simulink model "EV_powertrain"  (R2020a)
settings: Solver=FixedStepAuto  StartTime=0.0  StopTime=120.0  RelTol=1e-3
values from neighbouring files (symbols this model uses):
  A = 1452*mm*1799*mm    (= 2.612148)    [Model_parameters.m]
  b_r = 4.924e-4*(Nm/rad)    (= 0.0004924)    [Model_parameters.m]
  C_d = 0.27    [Model_parameters.m]
  c_roll = 0.0125    [Model_parameters.m]
  g = 9.81*(meters/(sec^2))    (= 9.81)    [Model_parameters.m]
  J_r = 0.089*kg*meters^2    (= 0.089)    [Model_parameters.m]
  K_rg = 10^13*(Newton/meters)    (= 10000000000000)    [Model_parameters.m]
  lambda_pm = 0.1039*Weber    (= 0.1039)    [Model_parameters.m]
  M = 1300*kg    (= 1300)    [Model_parameters.m]
  P_2_0 = 0    [Model_parameters.m]
  P_4_0 = 0    [Model_parameters.m]
  pp = 4    [Model_parameters.m]
  pwm_switch_period = 2e-5    (= 2e-05)    [Model_parameters.m]
  r_g = 9.7*r_r    (= 0.097)    [Model_parameters.m]
  r_r = 1*cm    (= 0.01)    [Model_parameters.m]
  r_w = 32*cm    (= 0.32)    [Model_parameters.m]
  rho = 1.225*(kg/(meters^3))    (= 1.225)    [Model_parameters.m]
  slope_out = tan(-0.3*[ 0  0  0  0  0  0  0  0  0  0 0]*degrees)    [Model_parameters.m]
  x_5_0 = 0    [Model_parameters.m]
  x_in = [ 0 12 38 65 78 100 112 138 165 178 200]*meters    [Model_parameters.m]
libraries: eePwmGenerator x3, simulink x1, autolibdatasheetbattery x1, autolibmotorctrlr x1, autolibpmsmexterior x1, autolibinverter x1
settings Model: Creator=giaco  LastModifiedBy=annac

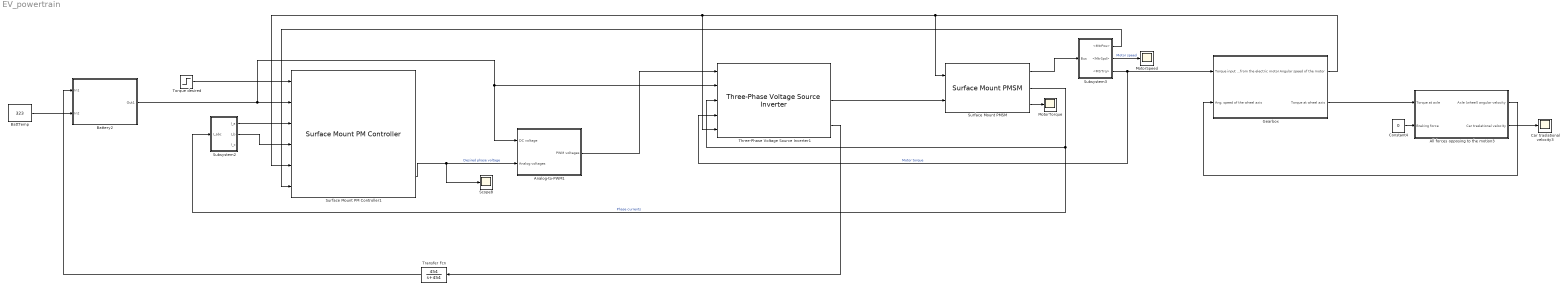
== system EV_powertrain ==
  All forces opposing to the motion3 : Subsystem
  Analog-to-PWM1 : Subsystem
  BattTemp : Constant  Value=323
  Battery2 : Subsystem
  Car traslational velocity3 : Scope
  Constant4 : Constant  Value=0
  Gearbox : Subsystem
  MotorSpeed : Scope
  MotorTorque : Scope
  Scope8 : Scope
  Subsystem2 : Subsystem
  Subsystem3 : Subsystem
  Surface Mount PM Controller1 : autolibmotorctrlr/Surface Mount PM Controller  control_type=Torque Control  Rs=R_s  Ldq=L_s  Ld=0.000391  Lq=0.000391  lambda_pm=lambda_pm  PolePairs=pp  Mechanical=[J_r, b_r, 0]  T_max=max_torque_motor  bp=10  T_mtpa=[0 6.66669841797461 13.3335873347246 20.0008572036754 26.6686983876046 33.3373011134498 40.0068554272732 46.6775511494351 53.3495778300274 60.0231247046184]  id_mtpa=[0 -0.0287202961052195 -0.114874619738106 -0.258443284350566 -0.459393504010068 -0.717679430800711 -1.03324220704656 -1.40601003221657 -1.8358982443354 -2.32280941568585]  iq_mtpa=[0 9.30574388067393 18.6112218818157 27.9161683137524 37.220317866163 46.5234057968387 55.8251681193482 65.12534178925 74.4236648884977 83.7198768076925]  idq_limits=401.0266  EV_current=500000  Tst=T_sample_torque_control  Kp_d=1178.7256  Kp_q=1178.7256  Ki=628318.5307  EV_motion=[20, 4, 0.8]  EV_sf=100  ba=50  Ksa=10  Kisa=0.05  Ksf=10  Jcomp=J_r  Fv=b_r  Fs=0  param_loss=Single efficiency measurement  eff=inverter_efficiency  w_loss_bp=[0 200 400 600 800 1000]  T_loss_bp=[0 25 50 75 100]  losses_table=[100 100 100 100 100;100 150 200 250 300;100 200 300 400 500;100 250 400 550 700;100 300 500 700 900;100 350 600 850 1100]  w_eff_bp=[200 400 600 800 1000]  T_eff_bp=[25 50 75 100]  efficiency_table=[96.2 98.1 98.7 99;98.1 99 99.4 99.5;98.7 99.4 99.6 99.7;99 99.5 99.7 99.8;99.2 99.6 99.7 99.8]  x_w_bp=[-1000 -800 -600 -400 -200 200 400 600 800 1000]  x_T_bp=[-100 -75 -50 -25 25 50 75 100]  x_losses_mat=[200.400801603196 225.67703109328 200.803212851408 201.612903225806 199.999999999997 200 225 200;160.320641282556 180.541624874624 201.005025125625 202.020202020203 200 200 180 160;180.541624874624 180.722891566267 181.086519114686 197.568389057748 194.999999999999 179.999999999997 180 180;201.005025125625 181.086519114686 202.020202020203 193.67991845056 190 200 179.999999999997 200;202.020202020203 197.568389057748 193.67991845056 197.505197505197 190 190 194.999999999999 200;200 194.999999999999 190 190 197.505197505197 193.67991845056 197.568389057748 202.020202020203;200 179.999999999997 200 190 193.67991845056 202.020202020203 181.086519114686 201.005025125625;180 180 179.999999999997 194.999999999999 197.568389057748 181.086519114686 180.722891566267 180.541624874624;160 180 200 200 202.020202020203 201.005025125625 180.541624874624 160.320641282556;200 225 200 199.999999999997 201.612903225806 200.803212851408 225.67703109328 200.400801603196]  Tsm=5e-4
      settings: SourceProductBaseCode=PW
  Surface Mount PMSM : autolibpmsmexterior/Surface Mount PMSM  port_config=Speed  sim_type=Continuous  Ts=0.001  FilePath=E:\Sandbox\Bauto\Work\surfacepmsm_motordata.m  P=pp  Rs=R_s  Ldq_=L_s  KConstText=Permanent flux linkage constant (lambda_pm):  lambda_pm=lambda_pm  Ke=159.9771  Kt=1.323  mechanical=[0.0027, 4.924e-4, 0]  idq0=[0 0]  theta_init=0  omega_init=0  KConst=lambda_pm  lambda_pm_calc=lambda_pm  RefBlkName='autolibpmsmexterior/Surface Mount PMSM'  aMode=1  Ldq="[0.000391    0.000391]"
      settings: SourceProductBaseCode=PW,MT,VE,VP
  Three-Phase Voltage Source Inverter1 : autolibinverter/Three-Phase Voltage Source Inverter  InvrtrTmpInpEnbl=off  enable_hdl=off  model_type=Switch inputs  fs=10000  w_eff_bp=[-1000 -500 0 500 1000]  n1=128  T_eff_bp=[-200 -100 0 100 200]  Temp_eff_bp=[213.15 293.15 373.15]  n2=128  ploss_table=[1 0.999 0.989 0.997 0.996;0.995 0.994 0.993 0.992 0.991;0.990 0.989 0.988 0.987 0.986;0.985 0.984 0.983 0.982 0.981;0.980 0.979 0.978 0.977 0.976]  ploss_table_3d=cat(3,0.95*[1 0.999 0.989 0.997 0.996;0.995 0.994 0.993 0.992 0.991;0.990 0.989 0.988 0.987 0.986;0.985 0.984 0.983 0.982 0.981;0.980 0.979 0.978 0.977 0.976],[1 0.999 0.989 0.997 0.996;0.995 0.994 0.993 0.992 0.991;0.990 0.989 0.988 0.987 0.986;0.985 0.984 0.983 0.982 0.981;0.980 0.979 0.978 0.977 0.976],0.92*[1 0.999 0.989 0.997 0.996;0.995 0.994 0.993 0.992 0.991;0.990 0.989 0.988 0.987 0.986;0.985 0.984 0.983 0.982 0.981;0.980 0.979 0.978 0.977 0.976])  preExtrapFlag=off  u1max=1000  u1min=-1000  u2max=200  u2min=-200  intPrec=23  RefBlkName='autolibmappedmotor/Mapped Motor'  CalLossMapData={'BaseCageProjectFileName','';'BaseMbcProjectFileName','';'TaskName','Calibrate Inverter Loss Map';'ChildTasks',{{'DataName','';'TaskName','Import Loss Data'},{'TaskName','Generate Response Models'},{'TaskName','Generate Calibration'},{'TaskName','Update Block Parameters'}}}  CalLossWithTempMapData={}
      settings: SourceProductBaseCode=PW,MT,VE,VP
  Torque desired : Step  Time=0.2  After=200  SampleTime=0
  Transfer Fcn : TransferFcn  Numerator=[454]  Denominator=[1 454]
  wires:
  Surface Mount PM Controller1/3 -> Scope8/1, Analog-to-PWM1/2(Analog voltages)  "Desired phase voltage"
  Torque desired/1 -> Surface Mount PM Controller1/1
  Analog-to-PWM1/1(PWM voltages) -> Three-Phase Voltage Source Inverter1/1
  Battery2/1(Out1) -> Analog-to-PWM1/1(DC voltage), Three-Phase Voltage Source Inverter1/2, Surface Mount PM Controller1/2
  Surface Mount PMSM/2 -> Three-Phase Voltage Source Inverter1/3, Subsystem2/1(I_abc)  "Phase currents"
  Surface Mount PMSM/1 -> Subsystem3/1(Bus)
  Subsystem3/3(<MtrTrq>) -> Gearbox/1(Torque input from the electric motor), Three-Phase Voltage Source Inverter1/4  "Motor torque"
  Three-Phase Voltage Source Inverter1/2 -> Surface Mount PMSM/2
  Subsystem3/1(<MtrPos>) -> Surface Mount PM Controller1/6
  Subsystem2/1(I_a) -> Surface Mount PM Controller1/3
  Subsystem2/2(I_b) -> Surface Mount PM Controller1/4
  Gearbox/1(Angular speed of the motor) -> Surface Mount PMSM/1, Three-Phase Voltage Source Inverter1/5, Surface Mount PM Controller1/5
  Constant4/1 -> All forces opposing to the motion3/2(Braking force)
  All forces opposing to the motion3/2(Car traslational velocity) -> Car traslational velocity3/1
  Gearbox/2(Torque at wheel axis) -> All forces opposing to the motion3/1(Torque at axle)
  All forces opposing to the motion3/1(Axle (wheel) angular velocity) -> Gearbox/2(Ang. speed of the wheel axis)
  BattTemp/1 -> Battery2/2(In2)
  Three-Phase Voltage Source Inverter1/3 -> Transfer Fcn/1
  Transfer Fcn/1 -> Battery2/1(In1)
  Surface Mount PMSM/3 -> MotorTorque/1
  Subsystem3/2(<MtrSpd>) -> MotorSpeed/1  "Motor speed"

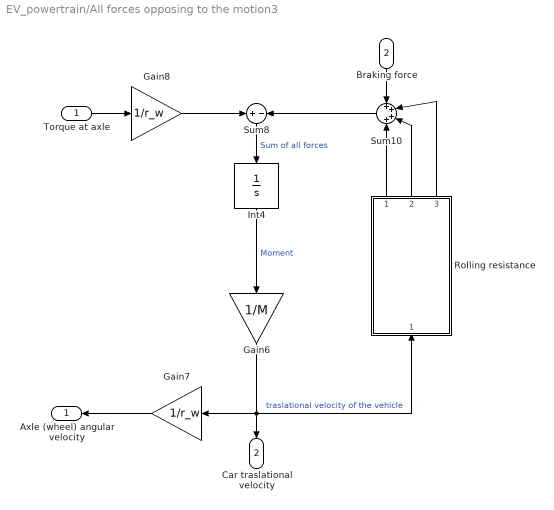
== system EV_powertrain/All forces opposing to the motion3 ==
  Torque at axle : Inport
  Braking force : Inport  Port=2
  Gain6 : Gain  Gain=1/M  SaturateOnIntegerOverflow=on  OutDataTypeStr=Inherit: Same as input  ParamDataTypeStr=Inherit: Same as input
  Gain7 : Gain  Gain=1/r_w  SaturateOnIntegerOverflow=on  OutDataTypeStr=Inherit: Same as input  ParamDataTypeStr=Inherit: Same as input
  Gain8 : Gain  Gain=1/r_w  SaturateOnIntegerOverflow=on  OutDataTypeStr=Inherit: Same as input  ParamDataTypeStr=Inherit: Same as input
  Int4 : Integrator  InitialCondition=P_4_0
  Rolling resistance : Subsystem
  Sum10 : Sum  Inputs=++++  InputSameDT=on  SaturateOnIntegerOverflow=on  OutDataTypeStr=Inherit: Same as first input
  Sum8 : Sum  Inputs=+|-  InputSameDT=on  SaturateOnIntegerOverflow=on  OutDataTypeStr=Inherit: Same as first input
  Axle (wheel) angular velocity : Outport  VectorParamsAs1DForOutWhenUnconnected=off
  Car traslational velocity : Outport  Port=2  VectorParamsAs1DForOutWhenUnconnected=off
  wires:
  Gain7/1 -> Axle (wheel) angular velocity/1
  Gain8/1 -> Sum8/1
  Sum8/1 -> Int4/1  "Sum of all forces"
  Gain6/1 -> Gain7/1, Rolling resistance/1(Traslational velocity), Car traslational velocity/1  "traslational velocity of the vehicle"
  Int4/1 -> Gain6/1  "Moment"
  Sum10/1 -> Sum8/2
  Torque at axle/1 -> Gain8/1
  Braking force/1 -> Sum10/1
  Rolling resistance/1(Rolling res) -> Sum10/4
  Rolling resistance/2("  Road slope") -> Sum10/3
  Rolling resistance/3(" Drag Force") -> Sum10/2

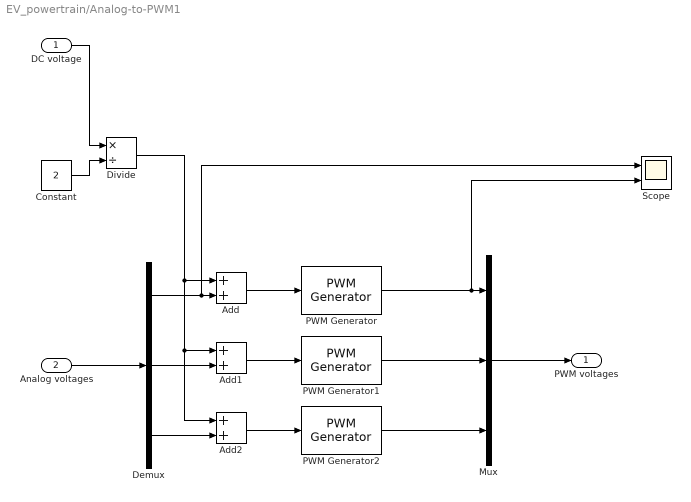
== system EV_powertrain/Analog-to-PWM1 ==
  DC voltage : Inport
  Analog voltages : Inport  Port=2
  Add : Sum
  Add1 : Sum
  Add2 : Sum
  Constant : Constant  Value=2
  Demux : Demux  Outputs=3
  Divide : Product  Inputs=*/
  Mux : Mux  Inputs=3
  PWM Generator : eePwmGenerator/PWM Generator  CarrCount=Up  Tper=0.02  Ts=pwm_switch_period
  PWM Generator1 : eePwmGenerator/PWM Generator  CarrCount=Up  Tper=0.02  Ts=pwm_switch_period
  PWM Generator2 : eePwmGenerator/PWM Generator  CarrCount=Up  Tper=0.02  Ts=pwm_switch_period
  Scope : Scope  NumInputPorts=2
  PWM voltages : Outport
  wires:
  Demux/1 -> Scope/1, Add/2
  PWM Generator/1 -> Scope/2, Mux/1
  PWM Generator2/1 -> Mux/3
  Add1/1 -> PWM Generator1/1
  Demux/2 -> Add1/2
  PWM Generator1/1 -> Mux/2
  Add/1 -> PWM Generator/1
  Add2/1 -> PWM Generator2/1
  Demux/3 -> Add2/2
  Analog voltages/1 -> Demux/1
  Mux/1 -> PWM voltages/1
  Constant/1 -> Divide/2
  DC voltage/1 -> Divide/1
  Divide/1 -> Add2/1, Add1/1, Add/1

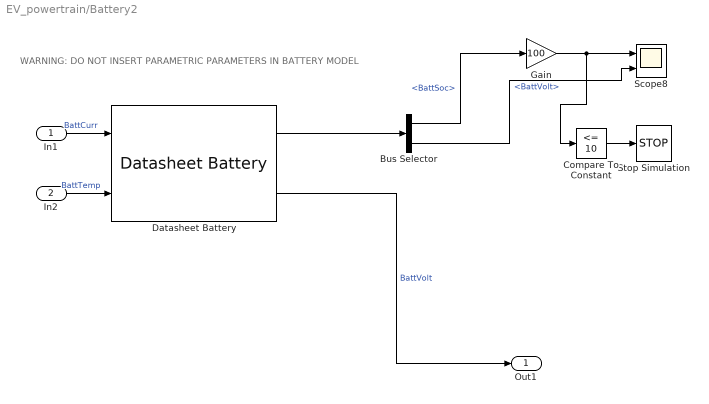
== system EV_powertrain/Battery2 ==
  note: WARNING: DO NOT INSERT PARAMETRIC PARAMETERS IN BATTERY MODEL
  In1 : Inport
  In2 : Inport  Port=2
  Bus Selector : BusSelector  OutputSignals=BattSoc,BattVolt
  Compare To Constant : simulink/Logic and Bit Operations/Compare To Constant  relop=<=  const=10  OutDataTypeStr=boolean
  Datasheet Battery : autolibdatasheetbattery/Datasheet Battery  CapacityCtrl=Parameter  OutputVlt=Unfiltered  BattChargeMax=100  Em=[2.8 3.228 3.284 3.361 3.408 3.427 3.472 3.477 3.493 3.504 3.516 3.528 3.537 3.545 3.555 3.561 3.566 3.576 3.587 3.589 3.594 3.6 3.608 3.61 3.616 3.619 3.626 3.632 3.637 3.64 3.645 3.646 3.652 3.655 3.658 3.661 3.664 3.668 3.673 3.678 3.68 3.681 3.686 3.692 3.699 3.702 3.705 3.71 3.717 3.723 3.728 3.733 3.735 3.742 3.749 3.755 3.761 3.768 3.773 3.78 3.791 3.798 3.798 3.814 3.818 3.825 3.841 3.846 3.855 3.863 3.877 3.885 3.894 3.907 3.919 3.926 3.935 3.944 3.954 3.964 3.974 3.988 3.998 4.014 4.029 4.034 4.047 4.065 4.074 4.086 4.097 4.131 4.126 4.138 4.15 4.18 4.174 4.187 4.207 4.231 4.221]  CapLUTBp=[0 0.01 0.02 0.03 0.04 0.05 0.06 0.07 0.08 0.09 0.1 0.11 0.12 0.13 0.14 0.15 0.16 0.17 0.18 0.19 0.2 0.21 0.22 0.23 0.24 0.25 0.26 0.27 0.28 0.29 0.3 0.31 0.32 0.33 0.34 0.35 0.36 0.37 0.38 0.39 0.4 0.41 0.42 0.43 0.44 0.45 0.46 0.47 0.48 0.49 0.5 0.51 0.52 0.53 0.54 0.55 0.56 0.57 0.58 0.59 0.6 0.61 0.62 0.63 0.64 0.65 0.66 0.67 0.68 0.69 0.7 0.71 0.72 0.73 0.74 0.75 0.76 0.77 0.78 0.79 0.8 0.81 0.82 0.83 0.84 0.85 0.86 0.87 0.88 0.89 0.9 0.91 0.92 0.93 0.94 0.95 0.96 0.97 0.98 0.99 1]  RInt=[0.008846 0.009319 0.009027 0.00847 0.01032 0.01314;0.006389 0.006554 0.005553 0.005525 0.006043 0.007805;0.004364 0.004101 0.00406 0.003452 0.003846 0.004517;0.002031 0.002563 0.002532 0.00246 0.002716 0.003047;0.001443 0.001825 0.001795 0.001778 0.001924 0.002234;0.0005603 0.0007192 0.0006887 0.0007557 0.0007355 0.001014;0.001028 0.001338 0.001 0.001536 0.001546 0.002789]  BattTempBp=[243.1 253.1 263.1 273.1 283.1 298.1 313.1]  CapSOCBp=[0 0.2 0.4 0.6 0.8 1]  Ns=143  Np=1  BattCapInit=100  Tc=1/1000  Vinit=4.221  RefBlkName='autolibdatasheetbattery/Datasheet Battery'
      settings: SourceProductBaseCode=PW
  Gain : Gain  Gain=100
  Scope8 : Scope  NumInputPorts=2
  Stop Simulation : Stop
  Out1 : Outport  VectorParamsAs1DForOutWhenUnconnected=off
  wires:
  Compare To Constant/1 -> Stop Simulation/1
  Gain/1 -> Scope8/1, Compare To Constant/1
  In2/1 -> Datasheet Battery/2  "BattTemp"
  Datasheet Battery/1 -> Bus Selector/1
  Datasheet Battery/2 -> Out1/1  "BattVolt"
  In1/1 -> Datasheet Battery/1  "BattCurr"
  Bus Selector/2 -> Scope8/2  "<BattVolt>"
  Bus Selector/1 -> Gain/1  "<BattSoc>"

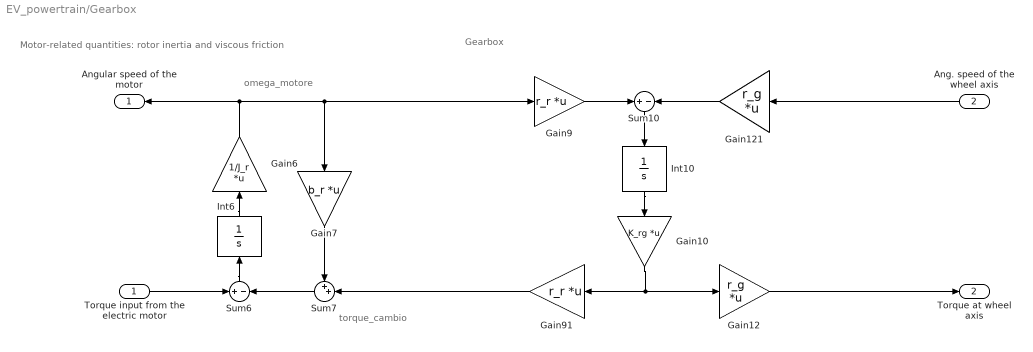
== system EV_powertrain/Gearbox ==
  note: omega_motore
  note: torque_cambio
  note: Motor-related quantities: rotor inertia and viscous friction
  note: Gearbox
  Torque input from the electric motor : Inport
  Ang. speed of the wheel axis : Inport  Port=2
  Gain10 : Gain  Gain=K_rg  Multiplication=Matrix(K*u)  SaturateOnIntegerOverflow=on  OutDataTypeStr=Inherit: Same as input  ParamDataTypeStr=Inherit: Same as input
  Gain12 : Gain  Gain=r_g  Multiplication=Matrix(K*u)  SaturateOnIntegerOverflow=on  OutDataTypeStr=Inherit: Same as input  ParamDataTypeStr=Inherit: Same as input
  Gain121 : Gain  Gain=r_g  Multiplication=Matrix(K*u)  SaturateOnIntegerOverflow=on  OutDataTypeStr=Inherit: Same as input  ParamDataTypeStr=Inherit: Same as input
  Gain6 : Gain  Gain=1/J_r  Multiplication=Matrix(K*u)  SaturateOnIntegerOverflow=on  OutDataTypeStr=Inherit: Same as input  ParamDataTypeStr=Inherit: Same as input
  Gain7 : Gain  Gain=b_r  Multiplication=Matrix(K*u)  SaturateOnIntegerOverflow=on  OutDataTypeStr=Inherit: Same as input  ParamDataTypeStr=Inherit: Same as input
  Gain9 : Gain  Gain=r_r  Multiplication=Matrix(K*u)  SaturateOnIntegerOverflow=on  OutDataTypeStr=Inherit: Same as input  ParamDataTypeStr=Inherit: Same as input
  Gain91 : Gain  Gain=r_r  Multiplication=Matrix(K*u)  SaturateOnIntegerOverflow=on  OutDataTypeStr=Inherit: Same as input  ParamDataTypeStr=Inherit: Same as input
  Int10 : Integrator  InitialCondition=x_5_0
  Int6 : Integrator  InitialCondition=P_2_0
  Sum10 : Sum  Inputs=+|-  InputSameDT=on  SaturateOnIntegerOverflow=on  OutDataTypeStr=Inherit: Same as first input
  Sum6 : Sum  Inputs=+|-  InputSameDT=on  SaturateOnIntegerOverflow=on  OutDataTypeStr=Inherit: Same as first input
  Sum7 : Sum  Inputs=++|  InputSameDT=on  SaturateOnIntegerOverflow=on  OutDataTypeStr=Inherit: Same as first input
  Angular speed of the motor : Outport  VectorParamsAs1DForOutWhenUnconnected=off
  Torque at wheel axis : Outport  Port=2  VectorParamsAs1DForOutWhenUnconnected=off
  wires:
  Torque input from the electric motor/1 -> Sum6/1
  Sum7/1 -> Sum6/2
  Sum6/1 -> Int6/1
  Int6/1 -> Gain6/1
  Gain7/1 -> Sum7/1
  Gain91/1 -> Sum7/2
  Gain6/1 -> Angular speed of the motor/1, Gain7/1, Gain9/1
  Gain121/1 -> Sum10/2
  Gain9/1 -> Sum10/1
  Int10/1 -> Gain10/1
  Sum10/1 -> Int10/1
  Gain10/1 -> Gain12/1, Gain91/1
  Gain12/1 -> Torque at wheel axis/1
  Ang. speed of the wheel axis/1 -> Gain121/1

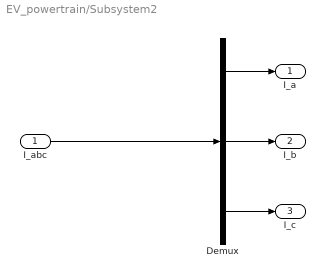
== system EV_powertrain/Subsystem2 ==
  I_abc : Inport
  Demux : Demux  Outputs=3
  I_a : Outport
  I_b : Outport  Port=2
  I_c : Outport  Port=3
  wires:
  I_abc/1 -> Demux/1
  Demux/1 -> I_a/1
  Demux/2 -> I_b/1
  Demux/3 -> I_c/1

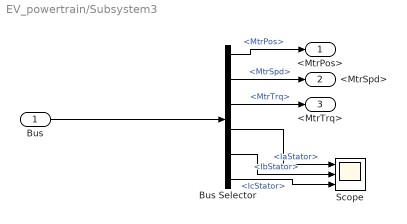
== system EV_powertrain/Subsystem3 ==
  Bus : Inport
  Bus Selector : BusSelector  OutputSignals=MtrPos,MtrSpd,MtrTrq,IaStator,IbStator,IcStator
  Scope : Scope  NumInputPorts=3
  <MtrPos> : Outport
  <MtrSpd> : Outport  Port=2
  <MtrTrq> : Outport  Port=3
  wires:
  Bus/1 -> Bus Selector/1
  Bus Selector/1 -> <MtrPos>/1  "<MtrPos>"
  Bus Selector/2 -> <MtrSpd>/1  "<MtrSpd>"
  Bus Selector/3 -> <MtrTrq>/1  "<MtrTrq>"
  Bus Selector/4 -> Scope/1  "<IaStator>"
  Bus Selector/5 -> Scope/2  "<IbStator>"
  Bus Selector/6 -> Scope/3  "<IcStator>"

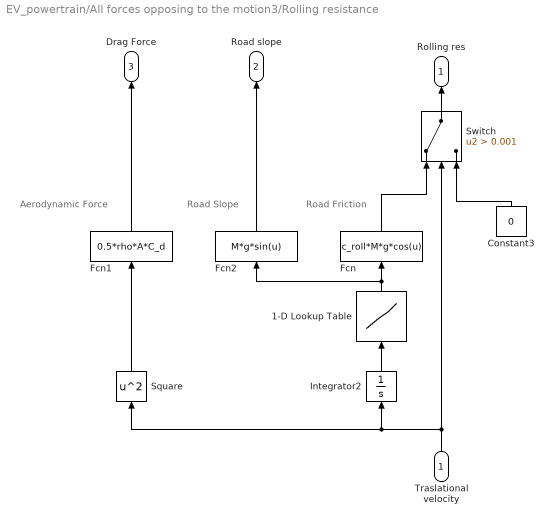
== system EV_powertrain/All forces opposing to the motion3/Rolling resistance ==
  note: Aerodynamic Force
  note: Road Friction
  note: Road Slope
  Traslational velocity : Inport
  1-D Lookup Table : Lookup_n-D  NumberOfTableDimensions=1  BreakpointsForDimension1=x_in  Table=slope_out  InternalRulePriority=Speed  RndMeth=Simplest  InputSameDT=on
  Constant3 : Constant  Value=0
  Fcn : Fcn  Expr=c_roll*M*g*cos(u)
  Fcn1 : Fcn  Expr=0.5*rho*A*C_d
  Fcn2 : Fcn  Expr=M*g*sin(u)
  Integrator2 : Integrator
  Square : Math  Operator=square  SignedPower=on  SaturateOnIntegerOverflow=on
  Switch : Switch  Criteria=u2 > Threshold  Threshold=0.001
  Rolling res : Outport
  "  Road slope" : Outport  Port=2
  " Drag Force" : Outport  Port=3
  wires:
  Switch/1 -> Rolling res/1
  Constant3/1 -> Switch/3
  Traslational velocity/1 -> Square/1, Integrator2/1, Switch/2
  Fcn2/1 -> "  Road slope"/1
  Fcn/1 -> Switch/1
  Integrator2/1 -> 1-D Lookup Table/1
  Fcn1/1 -> " Drag Force"/1
  Square/1 -> Fcn1/1
  1-D Lookup Table/1 -> Fcn2/1, Fcn/1
